simulink model "block_diagram"  (R2025a)
settings: Solver=VariableStepAuto  StartTime=0.0  StopTime=20.0  RelTol=1e-3
libraries: fuzblock x1
settings Model: Creator=HP  LastModifiedBy=HP

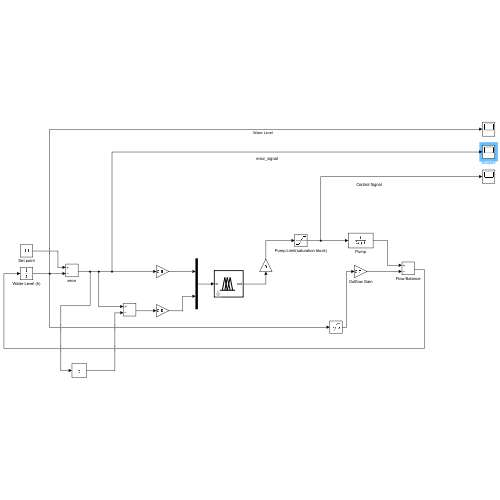
[thumbnail: Simulink's stored preview of the top-level diagram]
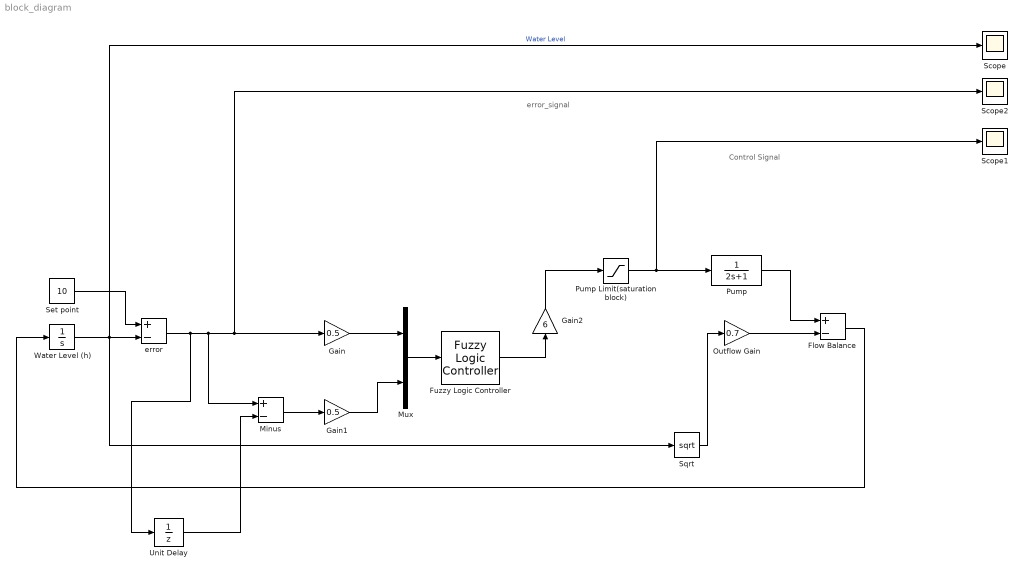
== system block_diagram ==
  note: Control Signal
  note: error_signal
  Flow Balance : Sum  Inputs=+-
  Fuzzy Logic Controller : fuzblock/Fuzzy Logic  Controller  FIS=tank  OutputSampleNumber=101  DataType=double  UseLookupTable=off  NumBreakpoints=10  FuzzifiedInputs=off  RuleFiringStrengths=off  RuleOutputs=off  AggregatedOutputs=off  SimulateUsing=Interpreted execution  OutOfRangeInputValueMessage=warning  NoRuleFiredMessage=warning  EmptyOutputFuzzySetMessage=warning
  Gain : Gain  Gain=0.5
  Gain1 : Gain  Gain=0.5
  Gain2 : Gain  Gain=6
  Minus : Sum  Inputs=+-
  Mux : Mux  Inputs=2
  Outflow Gain : Gain  Gain=0.7
  Pump : TransferFcn  Denominator=[2 1]
  Pump Limit(saturation block) : Saturate  UpperLimit=10  LowerLimit=-10
  Scope : Scope
      settings: ActiveDisplayYMinimum=-29.613512462946492  ActiveDisplayYMaximum=22.805923996543207
  Scope1 : Scope
      settings: ActiveDisplayYMinimum=-29.887069764395939  ActiveDisplayYMaximum=64.360182967764629
  Scope2 : Scope
      settings: ActiveDisplayYMinimum=-213.68820168175566  ActiveDisplayYMaximum=146.85878143119857  DataLoggingVariableName=ScopeData2
  Set point : Constant  Value=10
  Sqrt : Sqrt
  Unit Delay : UnitDelay  SampleTime=-1  HasFrameUpgradeWarning=on
  Water Level (h) : Integrator
  error : Sum  Inputs=+-
  wires:
  Sqrt/1 -> Outflow Gain/1
  Outflow Gain/1 -> Flow Balance/2
  error/1 -> Unit Delay/1, Minus/1, Gain/1, Scope2/1
  Pump Limit(saturation block)/1 -> Scope1/1, Pump/1
  Pump/1 -> Flow Balance/1
  Flow Balance/1 -> Water Level (h)/1
  Water Level (h)/1 -> Scope/1, Sqrt/1, error/2  "Water Level"
  Unit Delay/1 -> Minus/2
  Minus/1 -> Gain1/1
  Gain1/1 -> Mux/2
  Gain/1 -> Mux/1
  Gain2/1 -> Pump Limit(saturation block)/1
  Set point/1 -> error/1
  Fuzzy Logic Controller/1 -> Gain2/1
  Mux/1 -> Fuzzy Logic Controller/1
